simulink model "AUAV3_WITH_SLUGS_SENSOR_AND_CONTROLLER"  (Simulink 8.5)
settings: Solver=FixedStepDiscrete  StartTime=0.0  StopTime=10.0  FixedStep=T  RelTol=1e-3
PreLoadFcn:
  | T = 0.0025;
  | MavlinkBus;
  | 
  | % Baro Altitude Computation
  | % =========================
  | basePressure = 98192.64;
  | baseTemp = 288.215;
  | lapseRate = -0.00198122;
  | baseHeight = 0;
  | 
  | mcuInit
values from neighbouring files (symbols this model uses):
  apSampleTime = 0.01    [mcuInit.m]
  latlong_WP = 1    [mcuInit.m]
  mavlink_gps_raw_int_t = Simulink.Bus    [MavlinkBus.m]    (also in MavlinkBusMarcello.m)
  mavlink_raw_imu_t = Simulink.Bus    [MavlinkBus.m]    (also in MavlinkBusMarcello.m)
  mavlink_scaled_pressure_t = Simulink.Bus    [MavlinkBus.m]    (also in MavlinkBusMarcello.m)
  mavlink_sys_status_t = Simulink.Bus    [MavlinkBus.m]    (also in MavlinkBusMarcello.m)
  Xpoints = [0 0]    [mcuInit.m]
  Ypoints = [0 0]    [mcuInit.m]
  Zpoints = [0 0]    [mcuInit.m]
undefined symbols (not defined in the file or in its folder): A0, A14, A15, A2, A3, A5, A6, accBiasRateLimit, altLatLon, B0, bankCommandLimit, barAdjust, baroCutoff, baroCutTemp, C3, cubeAccelGain16405, cubeGyroGain16405, cubeMagGain16405, D0, D11, D13, D8, daLimit, data, daTrimMax, daTrimMin, deLimit, deTrimMax, deTrimMin, drLimit, drTrimMax, drTrimMin, dtLimit, dtTrimMax, dtTrimMin, F2, F3, G0, G15, gaind, GS_location, gyroBiasRateLimit, IC1max, IPStar, ISA_g, maxAcc, MaxDwnPthStar, maxDynPressure, maxEta, OC1max, P112, P127, P16, P21, P30, P31, P51, P64, P72, P75 ... (+39)
undefined symbols (not defined in the file): baroOffset, baroScale, barTGain1, barTGain2, barTMean1, barTMean2, bda, bde, bdr, bdt, bICda, bICde, bICdr, bICdt, derivativesConstant, lowRateSensorCutoff, mainSensorCutoff, mda, mde, mdr, mdt, mICda, mICde, mICdr, mICdt, pitotOffset, pitotScale, pitTGain1, pitTGain2, pitTMean1, pitTMean2, powerOffset, powerScale, pressureSensorCutoff, tempOffset, tempScale, vzCutoff, xCutoff, yCutoff
libraries: MCHP_Blockset x147, simulink x78, SLUGS_Library x31, aerolibconvert2 x6, aerolibutil x4, aerolibtransform2 x3, dspmtrx3 x2, aerolibobsolete x2
(part 7 of 12)

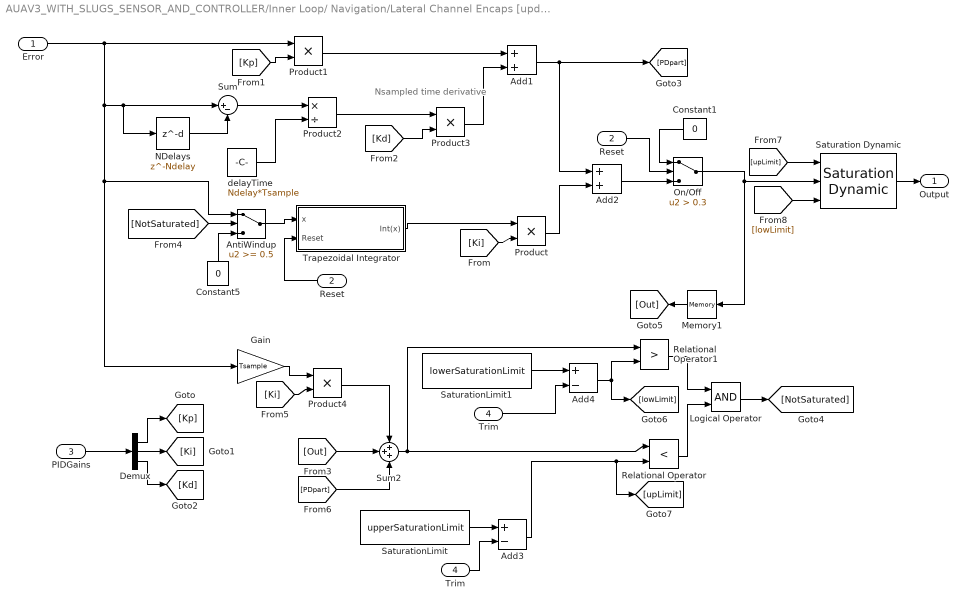
== system AUAV3_WITH_SLUGS_SENSOR_AND_CONTROLLER/Inner Loop/ Navigation/Lateral Channel Encaps [updated 4.28.16]/Lateral Channel/Roll Control [PID] ==
  note: Nsampled time derivative
  Error : Inport
  Reset : Inport  Port=2
  PIDGains : Inport  Port=3
  Trim : Inport  Port=4
  Add1 : Sum
  Add2 : Sum  OutDataTypeStr=single
  Add3 : Sum  Inputs=+-  OutDataTypeStr=single
  Add4 : Sum  Inputs=+-  OutDataTypeStr=single
  AntiWindup : Switch  Threshold=0.5
  Constant1 : Constant  Value=0  OutDataTypeStr=single
  Constant5 : Constant  Value=0  OutDataTypeStr=single
  Demux : Demux  Outputs=3
  Gain : Gain  Gain=Tsample
  Logical Operator : Logic  AllPortsSameDT=off  OutDataTypeStr=boolean
  Memory1 : Memory  InheritSampleTime=on
  NDelays : Delay  DelayLength=Ndelay  InputProcessing=Inherited  SampleTime=Tsample
  On/Off : Switch  Criteria=u2 > Threshold  Threshold=0.3
  Product{,1,3..4} (4 alike) : Product  RndMeth=Zero
  Product2 : Product  Inputs=*/  RndMeth=Zero
  Relational Operator : RelationalOperator  Operator=<  OutDataTypeStr=boolean
  Relational Operator1 : RelationalOperator  Operator=>  OutDataTypeStr=boolean
  "Reset " : InportShadow  Port=2
  Saturation Dynamic : simulink/Discontinuities/Saturation Dynamic  OutMin=[]  OutMax=[]  OutDataTypeStr=Inherit: Same as second input  OutDataType=fixdt(1, 16)  OutScaling=2^-10  DoSatur=off
  SaturationLimit : Constant  Value=upperSaturationLimit  OutDataTypeStr=single
  SaturationLimit1 : Constant  Value=lowerSaturationLimit  OutDataTypeStr=single
  Sum : Sum  Inputs=|+-
  Sum2 : Sum  Inputs=+++
  Trapezoidal Integrator : Subsystem  mask{T=Tsample}
      mask prompts: T "Sample Time"
  "Trim " : InportShadow  Port=4
  delayTime : Constant  Value=Ndelay*Tsample  OutDataTypeStr=single
  Output : Outport
  wires:
  On/Off/1 -> Memory1/1, Saturation Dynamic/2
  Constant1/1 -> On/Off/1
  "Reset "/1 -> On/Off/2
  Add2/1 -> On/Off/3
  [NotSaturated] -> AntiWindup/2
  Saturation Dynamic/1 -> Output/1
  Product2/1 -> Product3/1
  [Kd] -> Product3/2
  delayTime/1 -> Product2/2
  Sum/1 -> Product2/1
  NDelays/1 -> Sum/2
  [Kp] -> Product1/2
  Trapezoidal Integrator/1(Int(x)) -> Product/1
  [Ki] -> Product/2
  Error/1 -> Product1/1, Sum/1, NDelays/1, AntiWindup/1, Gain/1
  AntiWindup/1 -> Trapezoidal Integrator/1(x)
  Constant5/1 -> AntiWindup/3
  Demux/3 -> [Kd]
  Demux/2 -> [Ki]
  Demux/1 -> [Kp]
  PIDGains/1 -> Demux/1
  Memory1/1 -> [Out]
  Reset/1 -> Trapezoidal Integrator/2(Reset)
  Product1/1 -> Add1/1
  Product3/1 -> Add1/2
  Add1/1 -> [PDpart], Add2/1
  Product/1 -> Add2/2
  [PDpart] -> Sum2/3
  Product4/1 -> Sum2/1
  Gain/1 -> Product4/1
  [Ki] -> Product4/2
  Sum2/1 -> Relational Operator/1, Relational Operator1/1
  [Out] -> Sum2/2
  Add3/1 -> Relational Operator/2, [upLimit]
  Relational Operator/1 -> Logical Operator/2
  Relational Operator1/1 -> Logical Operator/1
  Logical Operator/1 -> [NotSaturated]
  Trim/1 -> Add3/2
  SaturationLimit/1 -> Add3/1
  Add4/1 -> Relational Operator1/2, [lowLimit]
  SaturationLimit1/1 -> Add4/1
  "Trim "/1 -> Add4/2
  [upLimit] -> Saturation Dynamic/1
  [lowLimit] -> Saturation Dynamic/3

== system AUAV3_WITH_SLUGS_SENSOR_AND_CONTROLLER/Inner Loop/ Navigation/Lateral Channel Encaps [updated 4.28.16]/Lateral Channel/Sideslip Compensation ==
  phi_m : Inport
  r_m : Inport  Port=2
  U_m : Inport  Port=3
  Enable : EnablePort  StatesWhenEnabling=reset
  Bank to Psi Dot : Subsystem  AncestorBlock=SLUGS_Library/Navigation/Bank to Psi Dot
  Constant : Constant  Value=0.3  OutDataTypeStr=single
  Low Pass : Subsystem
      mask Display:
      | droots([],'-a','a')
      | port_label('input',1,'a')
      | port_label('input',2,'u')
      | port_label('output',1,'y')
  Protect NaNs2 : Subsystem
  Subtract : Sum  Inputs=+-
  psi_dot to Bank : Subsystem  AncestorBlock=SLUGS_Library/Navigation/psi_dot to Bank
  bankComp : Outport  OutputWhenDisabled=reset  InitialOutput=0
  wires:
  Protect NaNs2/1(Out1) -> Low Pass/2(u)
  phi_m/1 -> Bank to Psi Dot/1(phi_c)
  r_m/1 -> Subtract/2
  U_m/1 -> Bank to Psi Dot/2(U_m), psi_dot to Bank/2(U_m)
  Bank to Psi Dot/1(psi_dot_c) -> Subtract/1  "coord turn"
  Subtract/1 -> psi_dot to Bank/1(psi_dot_c)  "turn rate error"
  psi_dot to Bank/1(phi_c) -> Protect NaNs2/1(In1)  "phi error"
  Low Pass/1(y) -> bankComp/1
  Constant/1 -> Low Pass/1(a)

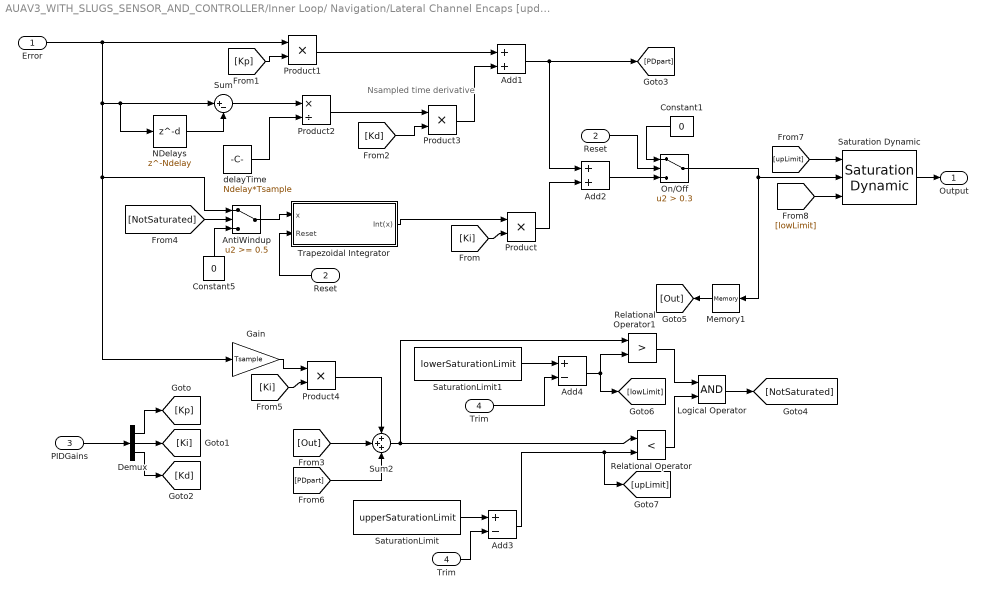
== system AUAV3_WITH_SLUGS_SENSOR_AND_CONTROLLER/Inner Loop/ Navigation/Lateral Channel Encaps [updated 4.28.16]/Lateral Channel/Yaw Damper [PID] ==
  note: Nsampled time derivative
  Error : Inport
  Reset : Inport  Port=2
  PIDGains : Inport  Port=3
  Trim : Inport  Port=4
  Add1 : Sum
  Add2 : Sum  OutDataTypeStr=single
  Add3 : Sum  Inputs=+-  OutDataTypeStr=single
  Add4 : Sum  Inputs=+-  OutDataTypeStr=single
  AntiWindup : Switch  Threshold=0.5
  Constant1 : Constant  Value=0  OutDataTypeStr=single
  Constant5 : Constant  Value=0  OutDataTypeStr=single
  Demux : Demux  Outputs=3
  Gain : Gain  Gain=Tsample
  Logical Operator : Logic  AllPortsSameDT=off  OutDataTypeStr=boolean
  Memory1 : Memory  InheritSampleTime=on
  NDelays : Delay  DelayLength=Ndelay  InputProcessing=Inherited  SampleTime=Tsample
  On/Off : Switch  Criteria=u2 > Threshold  Threshold=0.3
  Product{,1,3..4} (4 alike) : Product  RndMeth=Zero
  Product2 : Product  Inputs=*/  RndMeth=Zero
  Relational Operator : RelationalOperator  Operator=<  OutDataTypeStr=boolean
  Relational Operator1 : RelationalOperator  Operator=>  OutDataTypeStr=boolean
  "Reset " : InportShadow  Port=2
  Saturation Dynamic : simulink/Discontinuities/Saturation Dynamic  OutMin=[]  OutMax=[]  OutDataTypeStr=Inherit: Same as second input  OutDataType=fixdt(1, 16)  OutScaling=2^-10  DoSatur=off
  SaturationLimit : Constant  Value=upperSaturationLimit  OutDataTypeStr=single
  SaturationLimit1 : Constant  Value=lowerSaturationLimit  OutDataTypeStr=single
  Sum : Sum  Inputs=|+-
  Sum2 : Sum  Inputs=+++
  Trapezoidal Integrator : Subsystem  mask{T=Tsample}
      mask prompts: T "Sample Time"
  "Trim " : InportShadow  Port=4
  delayTime : Constant  Value=Ndelay*Tsample  OutDataTypeStr=single
  Output : Outport
  wires:
  On/Off/1 -> Memory1/1, Saturation Dynamic/2
  Constant1/1 -> On/Off/1
  "Reset "/1 -> On/Off/2
  Add2/1 -> On/Off/3
  [NotSaturated] -> AntiWindup/2
  Saturation Dynamic/1 -> Output/1
  Product2/1 -> Product3/1
  [Kd] -> Product3/2
  delayTime/1 -> Product2/2
  Sum/1 -> Product2/1
  NDelays/1 -> Sum/2
  [Kp] -> Product1/2
  Trapezoidal Integrator/1(Int(x)) -> Product/1
  [Ki] -> Product/2
  Error/1 -> Product1/1, Sum/1, NDelays/1, AntiWindup/1, Gain/1
  AntiWindup/1 -> Trapezoidal Integrator/1(x)
  Constant5/1 -> AntiWindup/3
  Demux/3 -> [Kd]
  Demux/2 -> [Ki]
  Demux/1 -> [Kp]
  PIDGains/1 -> Demux/1
  Memory1/1 -> [Out]
  Reset/1 -> Trapezoidal Integrator/2(Reset)
  Product1/1 -> Add1/1
  Product3/1 -> Add1/2
  Add1/1 -> [PDpart], Add2/1
  Product/1 -> Add2/2
  [PDpart] -> Sum2/3
  Product4/1 -> Sum2/1
  Gain/1 -> Product4/1
  [Ki] -> Product4/2
  Sum2/1 -> Relational Operator/1, Relational Operator1/1
  [Out] -> Sum2/2
  Add3/1 -> Relational Operator/2, [upLimit]
  Relational Operator/1 -> Logical Operator/2
  Relational Operator1/1 -> Logical Operator/1
  Logical Operator/1 -> [NotSaturated]
  Trim/1 -> Add3/2
  SaturationLimit/1 -> Add3/1
  Add4/1 -> Relational Operator1/2, [lowLimit]
  SaturationLimit1/1 -> Add4/1
  "Trim "/1 -> Add4/2
  [upLimit] -> Saturation Dynamic/1
  [lowLimit] -> Saturation Dynamic/3

== system AUAV3_WITH_SLUGS_SENSOR_AND_CONTROLLER/Inner Loop/ Navigation/Lateral Channel Encaps [updated 4.28.16]/Lateral Channel/psi_dot to Bank ==
  psi_dot_c : Inport
  U_m : Inport  Port=2
  Constant1 : Constant  Value=9.80665  OutDataTypeStr=single
  Divide : Product  Inputs=**/
  dsPIC_atan : Subsystem  AncestorBlock=SLUGS_Library/dsPIC_atan
  phi_c : Outport
  wires:
  Divide/1 -> dsPIC_atan/1(x)
  dsPIC_atan/1(atan(x)) -> phi_c/1
  Constant1/1 -> Divide/3
  U_m/1 -> Divide/2
  psi_dot_c/1 -> Divide/1

== system AUAV3_WITH_SLUGS_SENSOR_AND_CONTROLLER/Inner Loop/ Navigation/Lateral Channel Encaps [updated 4.28.16]/psi_dot_c Select logic1/Bank to Psi Dot ==
  phi_c : Inport
  U_m : Inport  Port=2
  Constant1 : Constant  Value=9.80665  OutDataTypeStr=single
  Divide : Product  Inputs=/*  OutDataTypeStr=single
  Divide1 : Product  OutDataTypeStr=single
  Protect NaNs : Subsystem
  Protect NaNs1 : Subsystem
  "[0 40]" : Saturate  UpperLimit=40  LowerLimit=0  SampleTime=.01
  bank Limit : Saturate  UpperLimit=bankCommandLimit  LowerLimit=-bankCommandLimit  SampleTime=.01
  dsPIC_tan : Subsystem  AncestorBlock=SLUGS_Library/dsPIC_tan
  psi_dot_c : Outport
  wires:
  "[0 40]"/1 -> Divide/1
  Divide/1 -> Divide1/2
  phi_c/1 -> Protect NaNs/1(In1)
  dsPIC_tan/1(tan(x)) -> Divide1/1
  Divide1/1 -> psi_dot_c/1
  Constant1/1 -> Divide/2
  U_m/1 -> Protect NaNs1/1(In1)
  bank Limit/1 -> dsPIC_tan/1(x)
  Protect NaNs/1(Out1) -> bank Limit/1
  Protect NaNs1/1(Out1) -> "[0 40]"/1

== system AUAV3_WITH_SLUGS_SENSOR_AND_CONTROLLER/Inner Loop/ Navigation/Longitudinal Channel Encaps [updated 4.28.16]/Longitudinal Channel/0.5 sec  tau for Turns ==
  In1 : Inport
  Constant : Constant  Value=T
  Constant1 : Constant  Value=f
  Embedded MATLAB Function : MATLAB Function  TreatAsAtomicUnit=on
  Out1 : Outport
  wires:
  Constant/1 -> Embedded MATLAB Function/2(T)
  Constant1/1 -> Embedded MATLAB Function/3(f)
  Embedded MATLAB Function/1(y) -> Out1/1
  In1/1 -> Embedded MATLAB Function/1(u)

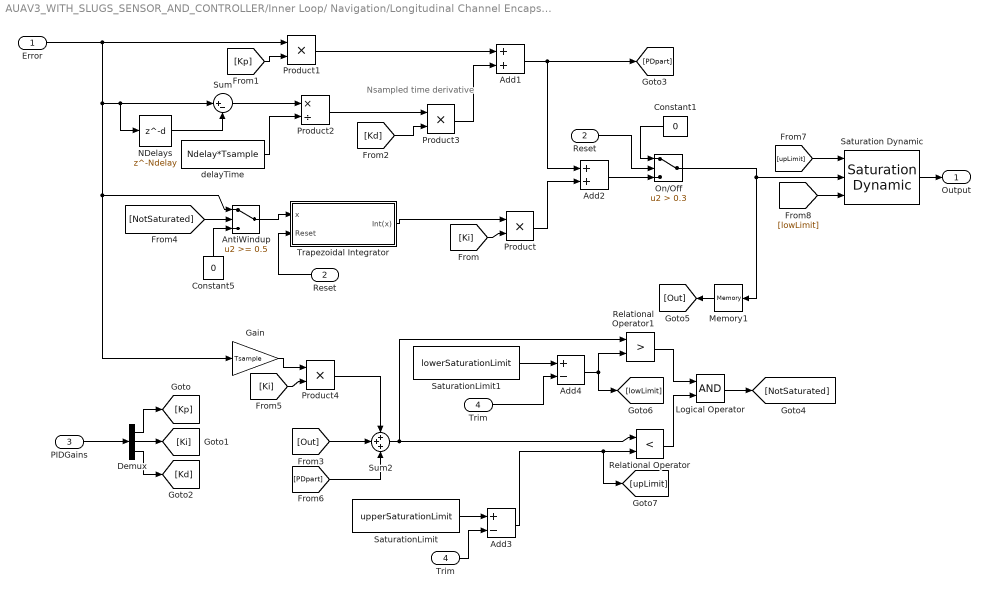
== system AUAV3_WITH_SLUGS_SENSOR_AND_CONTROLLER/Inner Loop/ Navigation/Longitudinal Channel Encaps [updated 4.28.16]/Longitudinal Channel/Airspeed Hold [PID] ==
  note: Nsampled time derivative
  Error : Inport
  Reset : Inport  Port=2
  PIDGains : Inport  Port=3
  Trim : Inport  Port=4
  Add1 : Sum
  Add2 : Sum  OutDataTypeStr=single
  Add3 : Sum  Inputs=+-  OutDataTypeStr=single
  Add4 : Sum  Inputs=+-  OutDataTypeStr=single
  AntiWindup : Switch  Threshold=0.5
  Constant1 : Constant  Value=0  OutDataTypeStr=single
  Constant5 : Constant  Value=0  OutDataTypeStr=single
  Demux : Demux  Outputs=3
  Gain : Gain  Gain=Tsample
  Logical Operator : Logic  AllPortsSameDT=off  OutDataTypeStr=boolean
  Memory1 : Memory  InheritSampleTime=on
  NDelays : Delay  DelayLength=Ndelay  InputProcessing=Inherited  SampleTime=Tsample
  On/Off : Switch  Criteria=u2 > Threshold  Threshold=0.3
  Product{,1,3..4} (4 alike) : Product  RndMeth=Zero
  Product2 : Product  Inputs=*/  RndMeth=Zero
  Relational Operator : RelationalOperator  Operator=<  OutDataTypeStr=boolean
  Relational Operator1 : RelationalOperator  Operator=>  OutDataTypeStr=boolean
  "Reset " : InportShadow  Port=2
  Saturation Dynamic : simulink/Discontinuities/Saturation Dynamic  OutMin=[]  OutMax=[]  OutDataTypeStr=Inherit: Same as second input  OutDataType=fixdt(1, 16)  OutScaling=2^-10  DoSatur=off
  SaturationLimit : Constant  Value=upperSaturationLimit  OutDataTypeStr=single
  SaturationLimit1 : Constant  Value=lowerSaturationLimit  OutDataTypeStr=single
  Sum : Sum  Inputs=|+-
  Sum2 : Sum  Inputs=+++
  Trapezoidal Integrator : Subsystem  mask{T=Tsample}
      mask prompts: T "Sample Time"
  "Trim " : InportShadow  Port=4
  delayTime : Constant  Value=Ndelay*Tsample  OutDataTypeStr=single
  Output : Outport
  wires:
  On/Off/1 -> Memory1/1, Saturation Dynamic/2
  Constant1/1 -> On/Off/1
  "Reset "/1 -> On/Off/2
  Add2/1 -> On/Off/3
  [NotSaturated] -> AntiWindup/2
  Saturation Dynamic/1 -> Output/1
  Product2/1 -> Product3/1
  [Kd] -> Product3/2
  delayTime/1 -> Product2/2
  Sum/1 -> Product2/1
  NDelays/1 -> Sum/2
  [Kp] -> Product1/2
  Trapezoidal Integrator/1(Int(x)) -> Product/1
  [Ki] -> Product/2
  Error/1 -> Product1/1, Sum/1, NDelays/1, AntiWindup/1, Gain/1
  AntiWindup/1 -> Trapezoidal Integrator/1(x)
  Constant5/1 -> AntiWindup/3
  Demux/3 -> [Kd]
  Demux/2 -> [Ki]
  Demux/1 -> [Kp]
  PIDGains/1 -> Demux/1
  Memory1/1 -> [Out]
  Reset/1 -> Trapezoidal Integrator/2(Reset)
  Product1/1 -> Add1/1
  Product3/1 -> Add1/2
  Add1/1 -> [PDpart], Add2/1
  Product/1 -> Add2/2
  [PDpart] -> Sum2/3
  Product4/1 -> Sum2/1
  Gain/1 -> Product4/1
  [Ki] -> Product4/2
  Sum2/1 -> Relational Operator/1, Relational Operator1/1
  [Out] -> Sum2/2
  Add3/1 -> Relational Operator/2, [upLimit]
  Relational Operator/1 -> Logical Operator/2
  Relational Operator1/1 -> Logical Operator/1
  Logical Operator/1 -> [NotSaturated]
  Trim/1 -> Add3/2
  SaturationLimit/1 -> Add3/1
  Add4/1 -> Relational Operator1/2, [lowLimit]
  SaturationLimit1/1 -> Add4/1
  "Trim "/1 -> Add4/2
  [upLimit] -> Saturation Dynamic/1
  [lowLimit] -> Saturation Dynamic/3

== system AUAV3_WITH_SLUGS_SENSOR_AND_CONTROLLER/Inner Loop/ Navigation/Longitudinal Channel Encaps [updated 4.28.16]/Longitudinal Channel/Height Error to Pitch  Command [PI] ==
  Error : Inport
  Reset : Inport  Port=2
  PIDGains : Inport  Port=3
  Trim : Inport  Port=4
  Add2 : Sum  OutDataTypeStr=single
  Add3 : Sum  Inputs=+-  OutDataTypeStr=single
  Add4 : Sum  Inputs=+-  OutDataTypeStr=single
  AntiWindup : Switch  Threshold=0.5
  Constant1 : Constant  Value=0  OutDataTypeStr=single
  Constant5 : Constant  Value=0  OutDataTypeStr=single
  Demux : Demux  Outputs=3
  Gain : Gain  Gain=Tsample
  Logical Operator : Logic  AllPortsSameDT=off  OutDataTypeStr=boolean
  Memory1 : Memory  InheritSampleTime=on
  On/Off : Switch  Criteria=u2 > Threshold  Threshold=0.3
  Product : Product  RndMeth=Zero
  Product1 : Product  RndMeth=Zero
  Product4 : Product  RndMeth=Zero
  Relational Operator : RelationalOperator  Operator=<  OutDataTypeStr=boolean
  Relational Operator1 : RelationalOperator  Operator=>  OutDataTypeStr=boolean
  "Reset " : InportShadow  Port=2
  Saturation Dynamic : simulink/Discontinuities/Saturation Dynamic  OutMin=[]  OutMax=[]  OutDataTypeStr=Inherit: Same as second input  OutDataType=fixdt(1, 16)  OutScaling=2^-10  DoSatur=off
  SaturationLimit : Constant  Value=upperSaturationLimit  OutDataTypeStr=single
  SaturationLimit1 : Constant  Value=lowerSaturationLimit  OutDataTypeStr=single
  Sum2 : Sum  Inputs=+++
  Terminator3 : Terminator
  Trapezoidal Integrator : Subsystem  mask{T=Tsample}
      mask prompts: T "Sample Time"
  "Trim " : InportShadow  Port=4
  Output : Outport
  wires:
  On/Off/1 -> Memory1/1, Saturation Dynamic/2
  Constant1/1 -> On/Off/1
  "Reset "/1 -> On/Off/2
  Add2/1 -> On/Off/3
  [lowLimit] -> Saturation Dynamic/3
  [upLimit] -> Saturation Dynamic/1
  "Trim "/1 -> Add4/2
  SaturationLimit1/1 -> Add4/1
  Add4/1 -> [lowLimit], Relational Operator1/2
  SaturationLimit/1 -> Add3/1
  Trim/1 -> Add3/2
  Logical Operator/1 -> [NotSaturated]
  Relational Operator1/1 -> Logical Operator/1
  Relational Operator/1 -> Logical Operator/2
  Add3/1 -> [upLimit], Relational Operator/2
  [Out] -> Sum2/2
  Sum2/1 -> Relational Operator1/1, Relational Operator/1
  [Ki] -> Product4/2
  Gain/1 -> Product4/1
  Product4/1 -> Sum2/1
  [PDpart] -> Sum2/3
  Product/1 -> Add2/2
  Product1/1 -> Add2/1, [PDpart]
  Reset/1 -> Trapezoidal Integrator/2(Reset)
  Memory1/1 -> [Out]
  PIDGains/1 -> Demux/1
  Demux/1 -> [Kp]
  Demux/2 -> [Ki]
  Constant5/1 -> AntiWindup/3
  AntiWindup/1 -> Trapezoidal Integrator/1(x)
  Error/1 -> Product1/1, Gain/1, AntiWindup/1
  [Ki] -> Product/2
  Trapezoidal Integrator/1(Int(x)) -> Product/1
  [Kp] -> Product1/2
  Saturation Dynamic/1 -> Output/1
  [NotSaturated] -> AntiWindup/2
  Demux/3 -> Terminator3/1

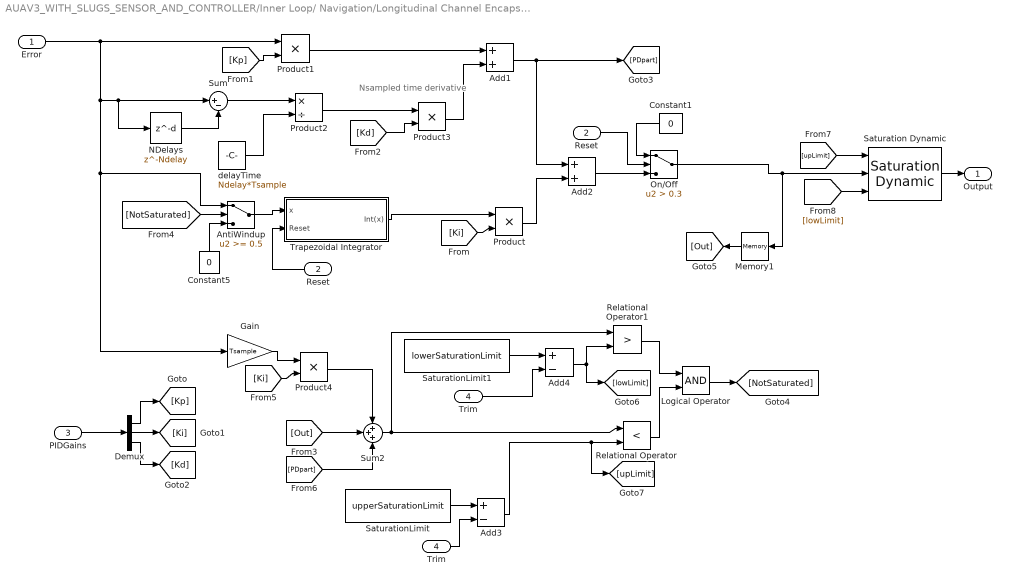
== system AUAV3_WITH_SLUGS_SENSOR_AND_CONTROLLER/Inner Loop/ Navigation/Longitudinal Channel Encaps [updated 4.28.16]/Longitudinal Channel/Pitch To Elevator [PID] ==
  note: Nsampled time derivative
  Error : Inport
  Reset : Inport  Port=2
  PIDGains : Inport  Port=3
  Trim : Inport  Port=4
  Add1 : Sum
  Add2 : Sum  OutDataTypeStr=single
  Add3 : Sum  Inputs=+-  OutDataTypeStr=single
  Add4 : Sum  Inputs=+-  OutDataTypeStr=single
  AntiWindup : Switch  Threshold=0.5
  Constant1 : Constant  Value=0  OutDataTypeStr=single
  Constant5 : Constant  Value=0  OutDataTypeStr=single
  Demux : Demux  Outputs=3
  Gain : Gain  Gain=Tsample
  Logical Operator : Logic  AllPortsSameDT=off  OutDataTypeStr=boolean
  Memory1 : Memory  InheritSampleTime=on
  NDelays : Delay  DelayLength=Ndelay  InputProcessing=Inherited  SampleTime=Tsample
  On/Off : Switch  Criteria=u2 > Threshold  Threshold=0.3
  Product{,1,3..4} (4 alike) : Product  RndMeth=Zero
  Product2 : Product  Inputs=*/  RndMeth=Zero
  Relational Operator : RelationalOperator  Operator=<  OutDataTypeStr=boolean
  Relational Operator1 : RelationalOperator  Operator=>  OutDataTypeStr=boolean
  "Reset " : InportShadow  Port=2
  Saturation Dynamic : simulink/Discontinuities/Saturation Dynamic  OutMin=[]  OutMax=[]  OutDataTypeStr=Inherit: Same as second input  OutDataType=fixdt(1, 16)  OutScaling=2^-10  DoSatur=off
  SaturationLimit : Constant  Value=upperSaturationLimit  OutDataTypeStr=single
  SaturationLimit1 : Constant  Value=lowerSaturationLimit  OutDataTypeStr=single
  Sum : Sum  Inputs=|+-
  Sum2 : Sum  Inputs=+++
  Trapezoidal Integrator : Subsystem  mask{T=Tsample}
      mask prompts: T "Sample Time"
  "Trim " : InportShadow  Port=4
  delayTime : Constant  Value=Ndelay*Tsample  OutDataTypeStr=single
  Output : Outport
  wires:
  On/Off/1 -> Memory1/1, Saturation Dynamic/2
  Constant1/1 -> On/Off/1
  "Reset "/1 -> On/Off/2
  Add2/1 -> On/Off/3
  [NotSaturated] -> AntiWindup/2
  Saturation Dynamic/1 -> Output/1
  Product2/1 -> Product3/1
  [Kd] -> Product3/2
  delayTime/1 -> Product2/2
  Sum/1 -> Product2/1
  NDelays/1 -> Sum/2
  [Kp] -> Product1/2
  Trapezoidal Integrator/1(Int(x)) -> Product/1
  [Ki] -> Product/2
  Error/1 -> Product1/1, Sum/1, NDelays/1, AntiWindup/1, Gain/1
  AntiWindup/1 -> Trapezoidal Integrator/1(x)
  Constant5/1 -> AntiWindup/3
  Demux/3 -> [Kd]
  Demux/2 -> [Ki]
  Demux/1 -> [Kp]
  PIDGains/1 -> Demux/1
  Memory1/1 -> [Out]
  Reset/1 -> Trapezoidal Integrator/2(Reset)
  Product1/1 -> Add1/1
  Product3/1 -> Add1/2
  Add1/1 -> [PDpart], Add2/1
  Product/1 -> Add2/2
  [PDpart] -> Sum2/3
  Product4/1 -> Sum2/1
  Gain/1 -> Product4/1
  [Ki] -> Product4/2
  Sum2/1 -> Relational Operator/1, Relational Operator1/1
  [Out] -> Sum2/2
  Add3/1 -> Relational Operator/2, [upLimit]
  Relational Operator/1 -> Logical Operator/2
  Relational Operator1/1 -> Logical Operator/1
  Logical Operator/1 -> [NotSaturated]
  Trim/1 -> Add3/2
  SaturationLimit/1 -> Add3/1
  Add4/1 -> Relational Operator1/2, [lowLimit]
  SaturationLimit1/1 -> Add4/1
  "Trim "/1 -> Add4/2
  [upLimit] -> Saturation Dynamic/1
  [lowLimit] -> Saturation Dynamic/3

== system AUAV3_WITH_SLUGS_SENSOR_AND_CONTROLLER/Inner Loop/ Navigation/Longitudinal Channel Encaps [updated 4.28.16]/Longitudinal Channel/Pitot Control End ==
  dyn P [Pa] : Inport
  H_m [m] : Inport  Port=2
  " 0.3 sec tau for high speeds" : Subsystem  mask(Tustin1stOrderLowpassAutoInitialCondition){f=1, T=T}
      mask prompts: f "Lowpass Frequency"; T "Sample Time"
      mask help: Takes a 3db rolloff frequency (in Hz, NOT radians/s) and a sample time. Performs a symbolic Tustin conversion and implements in a discrete filter. The initial output of the filter is set by the first sample.
      mask Help: Enter the desired 3db rolloff frequency in Hz and the sample time. Initial conditions are sampled automatically.
      mask Display: fprintf('%.2f Hz lowpass',f)
  Air Density from Height : Subsystem
  Compute Airspeed : Subsystem
  Protect NaN : Subsystem
  Schedule LPF : Switch  Criteria=u2 > Threshold  Threshold=0.3  OutDataTypeStr=single
  lowpass limit : simulink/Logic and Bit Operations/Compare To Constant  relop=<=  const=5  OutDataTypeStr=uint8  ZeroCross=off
  AirSpeed[m/s] : Outport
  wires:
  H_m [m]/1 -> Air Density from Height/1(h(m))
  Schedule LPF/1 -> AirSpeed[m/s]/1
  dyn P [Pa]/1 -> Compute Airspeed/1(Dyn P)
  Air Density from Height/1(rho (Kg/m^3)) -> Compute Airspeed/2(rho)
  Compute Airspeed/1(Airspeed m(s)) -> Protect NaN/1(In1)
  lowpass limit/1 -> Schedule LPF/2
  " 0.3 sec tau for high speeds"/1(Out1) -> Schedule LPF/3
  Protect NaN/1(Out1) -> " 0.3 sec tau for high speeds"/1(In1), lowpass limit/1, Schedule LPF/1

== system AUAV3_WITH_SLUGS_SENSOR_AND_CONTROLLER/Inner Loop/ Navigation/Longitudinal Channel Encaps [updated 4.28.16]/Longitudinal Channel/Protect NaNs ==
  In1 : Inport
  Integer Delay3 : Delay  DelayLength=1  InputProcessing=Inherited  SampleTime=T
  Relational Operator2 : RelationalOperator  Operator===  OutDataTypeStr=uint(8)
  Switch3 : Switch  Criteria=u2 > Threshold  Threshold=0.3  SampleTime=.01
  Out1 : Outport
  wires:
  Integer Delay3/1 -> Switch3/3
  Switch3/1 -> Out1/1, Integer Delay3/1
  In1/1 -> Relational Operator2/2, Relational Operator2/1, Switch3/1
  Relational Operator2/1 -> Switch3/2

== system AUAV3_WITH_SLUGS_SENSOR_AND_CONTROLLER/Inner Loop/ Navigation/Longitudinal Channel Encaps [updated 4.28.16]/Longitudinal Channel/Protect NaNs1 ==
  In1 : Inport
  Integer Delay3 : Delay  DelayLength=1  InputProcessing=Inherited  SampleTime=T
  Relational Operator2 : RelationalOperator  Operator===  OutDataTypeStr=uint(8)
  Switch3 : Switch  Criteria=u2 > Threshold  Threshold=0.3  SampleTime=.01
  Out1 : Outport
  wires:
  Integer Delay3/1 -> Switch3/3
  Switch3/1 -> Out1/1, Integer Delay3/1
  In1/1 -> Relational Operator2/2, Relational Operator2/1, Switch3/1
  Relational Operator2/1 -> Switch3/2

== system AUAV3_WITH_SLUGS_SENSOR_AND_CONTROLLER/Inner Loop/ Navigation/Longitudinal Channel Encaps [updated 4.28.16]/Longitudinal Channel/Protect NaNs2 ==
  In1 : Inport
  Integer Delay3 : Delay  DelayLength=1  InputProcessing=Inherited  SampleTime=T
  Relational Operator2 : RelationalOperator  Operator===  OutDataTypeStr=uint(8)
  Switch3 : Switch  Criteria=u2 > Threshold  Threshold=0.3  SampleTime=.01
  Out1 : Outport
  wires:
  Relational Operator2/1 -> Switch3/2
  In1/1 -> Switch3/1, Relational Operator2/1, Relational Operator2/2
  Switch3/1 -> Integer Delay3/1, Out1/1
  Integer Delay3/1 -> Switch3/3

== system AUAV3_WITH_SLUGS_SENSOR_AND_CONTROLLER/Inner Loop/ Navigation/Longitudinal Channel Encaps [updated 4.28.16]/Longitudinal Channel/Protect NaNs4 ==
  In1 : Inport
  Integer Delay3 : Delay  DelayLength=1  InputProcessing=Inherited  SampleTime=T
  Relational Operator2 : RelationalOperator  Operator===  OutDataTypeStr=uint(8)
  Switch3 : Switch  Criteria=u2 > Threshold  Threshold=0.3  SampleTime=.01
  Out1 : Outport
  wires:
  Relational Operator2/1 -> Switch3/2
  In1/1 -> Switch3/1, Relational Operator2/1, Relational Operator2/2
  Switch3/1 -> Integer Delay3/1, Out1/1
  Integer Delay3/1 -> Switch3/3

== system AUAV3_WITH_SLUGS_SENSOR_AND_CONTROLLER/Inner Loop/ Navigation/Longitudinal Channel Encaps [updated 4.28.16]/Longitudinal Channel/dsPIC_cos ==
  u : Inport
  Environment Controller1 : simulink/Signal Routing/Environment Controller
  Trigonometric Function : Trigonometry  Operator=cos
  myCos() apUtils.c [updated 5.1.16] : MCHP_Blockset/User Functions/C Function Call  ParseFilesChkbx=off  ListFunctions1=Custom Function  Function1=float myCos(float x)  AddHeaderDeclaration=off  Function1Type=when block is updated (default)  Fct1BlockIn=x  FctReturnBlockOut=on  DataCollected=0  ORDERING=None  SampleTime=-1  MCHP_MASTERLINK=|  PinDigitalInput=[]  PinDigitalOutput=[]  PinAnalogInput=[]
      | AUAV3_WITH_SLUGS_SENSOR_AND_CONTROLLER/Microchip Master
      | AUAV V3 Board
      | Busy Flag on D2 (RA6)
  cos(u) : Outport
  wires:
  u/1 -> Trigonometric Function/1, myCos() apUtils.c [updated 5.1.16]/1
  Environment Controller1/1 -> cos(u)/1
  myCos() apUtils.c [updated 5.1.16]/1 -> Environment Controller1/2
  Trigonometric Function/1 -> Environment Controller1/1

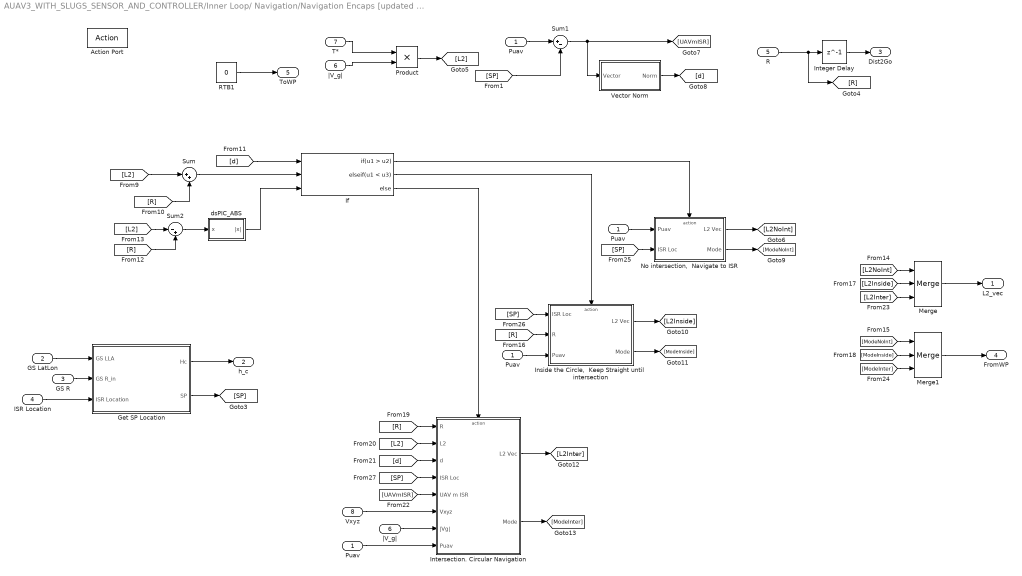
== system AUAV3_WITH_SLUGS_SENSOR_AND_CONTROLLER/Inner Loop/ Navigation/Navigation Encaps [updated 4.28.16]/Navigation/Circle Navigation ==
  Puav : Inport
  GS LatLon : Inport  Port=2
  GS R : Inport  Port=3
  ISR Location : Inport  Port=4
  R : Inport  Port=5
  |V_g| : Inport  Port=6
  T* : Inport  Port=7
  Vxyz : Inport  Port=8
  Action Port : ActionPort  ActionType=elseif
  Get SP Location : Subsystem
  If : If  NumInputs=3  IfExpression=u1 > u2  ElseIfExpressions=u1 < u3
  "Inside the Circle,  Keep Straight until  intersection" : Subsystem  TreatAsAtomicUnit=on
  Integer Delay : Delay  DelayLength=1  InputProcessing=Inherited
  Intersection. Circular Navigation : Subsystem  TreatAsAtomicUnit=on
  Merge : Merge  Inputs=3
  Merge1 : Merge  Inputs=3
  "No intersection,  Navigate to ISR" : Subsystem  TreatAsAtomicUnit=on
  Product : Product  OutDataTypeStr=single  RndMeth=Zero
  "Puav   " : InportShadow
  "Puav    " : InportShadow
  "Puav     " : InportShadow
  RTB1 : Constant  Value=0  OutDataTypeStr=uint8
  Sum : Sum  Inputs=|++
  Sum1 : Sum  Inputs=|+-
  Sum2 : Sum  Inputs=|-+
  Vector Norm : Subsystem  AncestorBlock=SLUGS_Library/Vector Norm
  dsPIC_ABS : Subsystem  AncestorBlock=SLUGS_Library/dsPIC_ABS
  "|V_g| " : InportShadow  Port=6
  L2_vec : Outport
  h_c : Outport  Port=2
  Dist2Go : Outport  Port=3
  FromWP : Outport  Port=4  InitialOutput=[1]
  ToWP : Outport  Port=5  InitialOutput=[1]
  wires:
  Merge1/1 -> FromWP/1
  R/1 -> [R], Integer Delay/1
  Integer Delay/1 -> Dist2Go/1
  ISR Location/1 -> Get SP Location/3(ISR Location)
  GS R/1 -> Get SP Location/2(GS R_in)
  GS LatLon/1 -> Get SP Location/1(GS LLA)
  Get SP Location/2(SP) -> [SP]
  Product/1 -> [L2]
  |V_g|/1 -> Product/2
  T*/1 -> Product/1
  RTB1/1 -> ToWP/1
  [L2] -> Sum/1
  [R] -> Sum/2
  "Puav   "/1 -> Sum1/1
  [SP] -> Sum1/2
  Sum1/1 -> Vector Norm/1(Vector), [UAVmISR]
  Vector Norm/1(Norm) -> [d]
  [d] -> If/1
  Sum/1 -> If/2
  [L2] -> Sum2/1
  [R] -> Sum2/2
  Sum2/1 -> dsPIC_ABS/1(x)
  dsPIC_ABS/1(|x|) -> If/3
  Merge/1 -> L2_vec/1
  If/1 -> "No intersection,  Navigate to ISR"/Action
  If/2 -> "Inside the Circle,  Keep Straight until  intersection"/Action
  If/3 -> Intersection. Circular Navigation/Action
  "Puav    "/1 -> "No intersection,  Navigate to ISR"/1(Puav)
  [SP] -> "No intersection,  Navigate to ISR"/2(ISR Loc)
  "No intersection,  Navigate to ISR"/1(L2 Vec) -> [L2NoInt]
  "No intersection,  Navigate to ISR"/2(Mode) -> [ModeNoInt]
  [L2NoInt] -> Merge/1
  [ModeNoInt] -> Merge1/1
  [SP] -> "Inside the Circle,  Keep Straight until  intersection"/1(ISR Loc)
  [R] -> "Inside the Circle,  Keep Straight until  intersection"/2(R)
  "Inside the Circle,  Keep Straight until  intersection"/1(L2 Vec) -> [L2Inside]
  "Inside the Circle,  Keep Straight until  intersection"/2(Mode) -> [ModeInside]
  [L2Inside] -> Merge/2
  [ModeInside] -> Merge1/2
  Puav/1 -> "Inside the Circle,  Keep Straight until  intersection"/3(Puav)
  Intersection. Circular Navigation/1(L2 Vec) -> [L2Inter]
  Intersection. Circular Navigation/2(Mode) -> [ModeInter]
  [R] -> Intersection. Circular Navigation/1(R)
  [L2] -> Intersection. Circular Navigation/2(L2)
  [d] -> Intersection. Circular Navigation/3(d)
  [SP] -> Intersection. Circular Navigation/4(ISR Loc)
  [UAVmISR] -> Intersection. Circular Navigation/5(UAV m ISR)
  Vxyz/1 -> Intersection. Circular Navigation/6(Vxyz)
  "|V_g| "/1 -> Intersection. Circular Navigation/7(|Vg|)
  [L2Inter] -> Merge/3
  [ModeInter] -> Merge1/3
  Get SP Location/1(Hc) -> h_c/1
  "Puav     "/1 -> Intersection. Circular Navigation/8(Puav)

== system AUAV3_WITH_SLUGS_SENSOR_AND_CONTROLLER/Inner Loop/ Navigation/Navigation Encaps [updated 4.28.16]/Navigation/Get 2D Groundspeed ==
  Vxyz : Inport  SampleTime=apSampleTime
  Vector Norm : Subsystem  AncestorBlock=SLUGS_Library/Vector Norm
  |V_g| : Outport
  wires:
  Vxyz/1 -> Vector Norm/1(Vector)
  Vector Norm/1(Norm) -> |V_g|/1

== system AUAV3_WITH_SLUGS_SENSOR_AND_CONTROLLER/Inner Loop/ Navigation/Navigation Encaps [updated 4.28.16]/Navigation/L2+ ==
  |V_g| : Inport
  L2_vec : Inport  Port=2
  Vxyz : Inport  Port=3
  T*(m) : Inport  Port=4
  Constant10 : Constant  Value=maxEta  OutDataTypeStr=single
  "Get Sin, Cos eta" : Subsystem
  L2+ : Subsystem
  Rad2Deg : Gain  Gain=180/pi
  Relational Operator : RelationalOperator  Operator=<=  OutDataTypeStr=boolean
  Subsystem : Subsystem
  Switch : Switch  Criteria=u2 > Threshold  Threshold=0.3
  dsPIC_ABS : Subsystem  AncestorBlock=SLUGS_Library/dsPIC_ABS
  dsPIC_atan2 : Subsystem  AncestorBlock=SLUGS_Library/dsPIC_atan2
  "if sin(eta) < 0 - maxAcc else                 maxAcc " : Subsystem
  "|V_g| " : InportShadow
  phi_c : Outport
  eta : Outport  Port=2
  wires:
  Vxyz/1 -> "Get Sin, Cos eta"/3(Vxyz)
  L2_vec/1 -> "Get Sin, Cos eta"/2(L2_vec)
  |V_g|/1 -> "Get Sin, Cos eta"/1(|V_g|)
  Switch/1 -> Subsystem/1(a_c)
  "if sin(eta) < 0 - maxAcc else                 maxAcc "/1(+ - maxAcc) -> Switch/3
  L2+/1(a_c) -> Switch/1
  Relational Operator/1 -> Switch/2
  Constant10/1 -> Relational Operator/2
  dsPIC_ABS/1(|x|) -> Relational Operator/1
  dsPIC_atan2/1(atan2(x,y)) -> dsPIC_ABS/1(x), Rad2Deg/1  "eta"
  "Get Sin, Cos eta"/2(cos(eta)) -> dsPIC_atan2/2(v)
  "Get Sin, Cos eta"/1(sin(eta)) -> "if sin(eta) < 0 - maxAcc else                 maxAcc "/1(sin(eta)), dsPIC_atan2/1(u), L2+/1(sin(eta))
  "|V_g| "/1 -> L2+/2(|V_g|)
  T*(m)/1 -> L2+/3(T*)
  Subsystem/1(phi_c) -> phi_c/1
  Rad2Deg/1 -> eta/1

== system AUAV3_WITH_SLUGS_SENSOR_AND_CONTROLLER/Inner Loop/ Navigation/Navigation Encaps [updated 4.28.16]/Navigation/Line Segment ==
  Puav : Inport
  MidLvl h_c : Inport  Port=2
  Action Port : ActionPort  ActionType=elseif
  Gain : Gain  Gain=-1
  Gain1 : Gain  Gain=-1
  "Puav " : InportShadow
  RTB : Constant  Value=0  OutDataTypeStr=uint8
  RTB1 : Constant  Value=0  OutDataTypeStr=uint8
  Vector Norm : Subsystem  AncestorBlock=SLUGS_Library/Vector Norm
  L2_vec : Outport
  h_c : Outport  Port=2
  Dist2Go : Outport  Port=3
  FromWP : Outport  Port=4  InitialOutput=[1]
  ToWP : Outport  Port=5  InitialOutput=[2]
  wires:
  RTB1/1 -> ToWP/1
  Gain1/1 -> Vector Norm/1(Vector)
  "Puav "/1 -> Gain1/1
  RTB/1 -> FromWP/1
  Vector Norm/1(Norm) -> Dist2Go/1
  MidLvl h_c/1 -> h_c/1
  Puav/1 -> Gain/1
  Gain/1 -> L2_vec/1

== system AUAV3_WITH_SLUGS_SENSOR_AND_CONTROLLER/Inner Loop/ Navigation/Navigation Encaps [updated 4.28.16]/Navigation/Minimum Turn Radius ==
  U_c : Inport
  Scale Factor : Inport  Port=2
  Constant1 : Constant  Value=maxAcc  OutDataTypeStr=single
  IC : InitialCondition  Value=1.5
  Product1 : Product  RndMeth=Zero
  Product2 : Product  RndMeth=Zero
  Product3 : Product  Inputs=*/  RndMeth=Zero
  "[1.5 10]" : Saturate  UpperLimit=10  LowerLimit=1.5
  R : Outport
  wires:
  IC/1 -> "[1.5 10]"/1
  "[1.5 10]"/1 -> Product2/1
  Product3/1 -> R/1
  Scale Factor/1 -> IC/1
  Product1/1 -> Product2/2
  Constant1/1 -> Product3/2
  Product2/1 -> Product3/1
  U_c/1 -> Product1/1, Product1/2

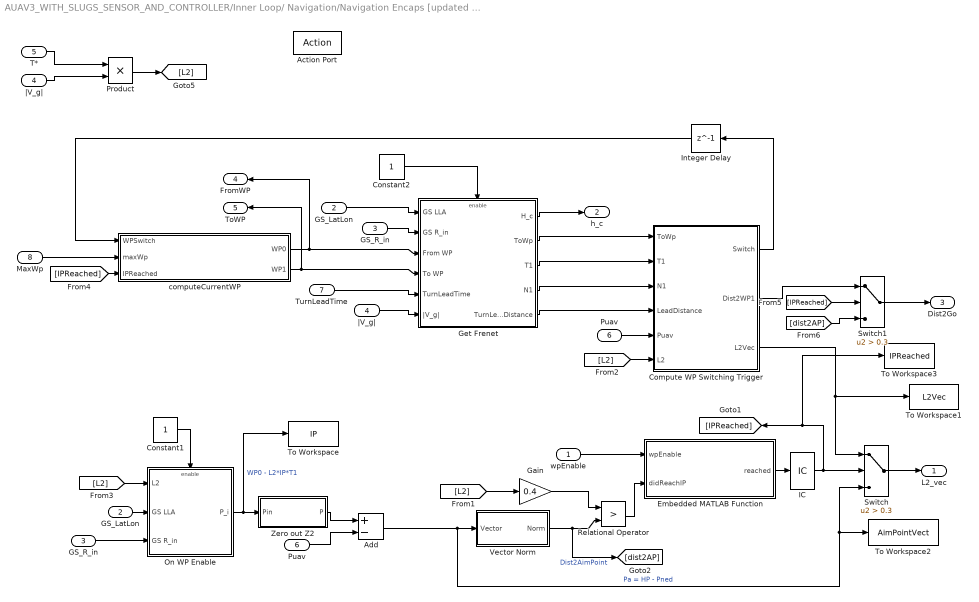
== system AUAV3_WITH_SLUGS_SENSOR_AND_CONTROLLER/Inner Loop/ Navigation/Navigation Encaps [updated 4.28.16]/Navigation/Normal WP  Navigation ==
  wpEnable : Inport
  GS_LatLon : Inport  Port=2
  GS_R_in : Inport  Port=3
  |V_g| : Inport  Port=4
  T* : Inport  Port=5
  Puav : Inport  Port=6
  TurnLeadTime : Inport  Port=7
  MaxWp : Inport  Port=8
  Action Port : ActionPort  ActionType=elseif
  Add : Sum  Inputs=+-
  Compute WP Switching Trigger : Subsystem
  Constant1 : Constant  OutDataTypeStr=boolean  SampleTime=0.01
  Constant2 : Constant  OutDataTypeStr=boolean  SampleTime=0.01
  Embedded MATLAB Function : MATLAB Function  TreatAsAtomicUnit=on
  "GS_LatLon " : InportShadow  Port=2
  "GS_R_in " : InportShadow  Port=3
  Gain : Gain  Gain=0.4
  Get Frenet : Subsystem
  IC : InitialCondition  Value=0
  Integer Delay : Delay  DelayLength=1  InitialCondition=1  InputProcessing=Inherited
  On WP Enable : Subsystem  TreatAsAtomicUnit=on
  Product : Product  OutDataTypeStr=single  RndMeth=Zero
  "Puav " : InportShadow  Port=6
  Relational Operator : RelationalOperator  Operator=>  OutDataTypeStr=boolean
  Switch : Switch  Criteria=u2 > Threshold  Threshold=0.3  ZeroCross=off
  Switch1 : Switch  Criteria=u2 > Threshold  Threshold=0.3  ZeroCross=off
  To Workspace : ToWorkspace  VariableName=IP  SampleTime=-1
  To Workspace1 : ToWorkspace  VariableName=L2Vec  SampleTime=-1
  To Workspace2 : ToWorkspace  VariableName=AimPointVect  SampleTime=-1
  To Workspace3 : ToWorkspace  VariableName=IPReached  SampleTime=-1
  Vector Norm : Subsystem  AncestorBlock=SLUGS_Library/Vector Norm
  Zero out Z2 : MATLAB Function  TreatAsAtomicUnit=on
  computeCurrentWP : MATLAB Function  TreatAsAtomicUnit=on
  "|V_g| " : InportShadow  Port=4
  L2_vec : Outport
  h_c : Outport  Port=2
  Dist2Go : Outport  Port=3
  FromWP : Outport  Port=4  InitialOutput=[1]
  ToWP : Outport  Port=5  InitialOutput=[2]
  wires:
  Get Frenet/1(H_c) -> h_c/1
  Constant2/1 -> Get Frenet/Enable
  Constant1/1 -> On WP Enable/Enable
  Integer Delay/1 -> computeCurrentWP/1(WPSwitch)
  [dist2AP] -> Switch1/3
  Switch1/1 -> Dist2Go/1
  Compute WP Switching Trigger/2(Dist2WP1) -> Switch1/1
  [IPReached] -> Switch1/2
  [IPReached] -> computeCurrentWP/3(IPReached)
  wpEnable/1 -> Embedded MATLAB Function/1(wpEnable)
  T*/1 -> Product/1
  |V_g|/1 -> Product/2
  Product/1 -> [L2]
  [L2] -> On WP Enable/1(L2)
  GS_LatLon/1 -> On WP Enable/2(GS LLA)
  GS_R_in/1 -> On WP Enable/3(GS R_in)
  On WP Enable/1(P_i) -> Zero out Z2/1(Pin), To Workspace/1  "WP0 - L2*IP*T1"
  Zero out Z2/1(P) -> Add/1
  Add/1 -> Vector Norm/1(Vector), Switch/3, To Workspace2/1  "Pa = HP - Pned"
  [L2] -> Gain/1
  Gain/1 -> Relational Operator/1
  Vector Norm/1(Norm) -> [dist2AP], Relational Operator/2  "Dist2AimPoint"
  Relational Operator/1 -> Embedded MATLAB Function/2(didReachIP)
  Switch/1 -> L2_vec/1
  Embedded MATLAB Function/1(reached) -> IC/1
  "GS_LatLon "/1 -> Get Frenet/1(GS LLA)
  "GS_R_in "/1 -> Get Frenet/2(GS R_in)
  Get Frenet/2(ToWp) -> Compute WP Switching Trigger/1(ToWp)
  Get Frenet/3(T1) -> Compute WP Switching Trigger/2(T1)
  Puav/1 -> Compute WP Switching Trigger/5(Puav)
  "Puav "/1 -> Add/2
  "|V_g| "/1 -> Get Frenet/6(|V_g|)
  TurnLeadTime/1 -> Get Frenet/5(TurnLeadTime)
  Get Frenet/5(TurnLeadDistance) -> Compute WP Switching Trigger/4(LeadDistance)
  Get Frenet/4(N1) -> Compute WP Switching Trigger/3(N1)
  Compute WP Switching Trigger/3(L2Vec) -> Switch/1, To Workspace1/1
  Compute WP Switching Trigger/1(Switch) -> Integer Delay/1
  computeCurrentWP/1(WP0) -> FromWP/1, Get Frenet/3(From WP)
  computeCurrentWP/2(WP1) -> ToWP/1, Get Frenet/4(To WP)
  MaxWp/1 -> computeCurrentWP/2(maxWp)
  [L2] -> Compute WP Switching Trigger/6(L2)
  IC/1 -> [IPReached], To Workspace3/1, Switch/2

== system AUAV3_WITH_SLUGS_SENSOR_AND_CONTROLLER/Inner Loop/ Navigation/Navigation Encaps [updated 4.28.16]/Navigation/RTB/Follow Mobile Navigation ==
  Mobile Location : Inport
  Follow Mobile? : Inport  Port=2
  MidLvl h_c : Inport  Port=3
  GS LatLon : Inport  Port=4
  GS R : Inport  Port=5
  Puav : Inport  Port=6
  Action Port : ActionPort  ActionType=then
  Compute Mobile Location : Subsystem  TreatAsAtomicUnit=on
  Constant : Constant  Value=[0 0 0]  OutDataTypeStr=single
  RTB : Constant  Value=0  OutDataTypeStr=uint8
  RTB1 : Constant  Value=0  OutDataTypeStr=uint8
  Simple Predictor : Subsystem
  Subtract : Sum  Inputs=+-
  Switch : Switch  Threshold=0.3
  To Workspace : ToWorkspace  VariableName=BP  SampleTime=-1
  Vector Norm : Subsystem  AncestorBlock=SLUGS_Library/Vector Norm
  Zero out Z1 : MATLAB Function  TreatAsAtomicUnit=on
  L2_vec : Outport
  h_c : Outport  Port=2
  Dist2Go : Outport  Port=3
  FromWP : Outport  Port=4  InitialOutput=[0]
  ToWP : Outport  Port=5  InitialOutput=[0]
  wires:
  RTB1/1 -> ToWP/1
  RTB/1 -> FromWP/1
  Vector Norm/1(Norm) -> Dist2Go/1
  Constant/1 -> Switch/3
  Compute Mobile Location/1(XYZ) -> Switch/1
  Follow Mobile?/1 -> Compute Mobile Location/Enable, Switch/2
  GS LatLon/1 -> Compute Mobile Location/2(GS LLA)
  GS R/1 -> Compute Mobile Location/3(GS R)
  Mobile Location/1 -> Compute Mobile Location/1("Lat, Lon")
  Simple Predictor/1(Predicted Bp) -> L2_vec/1
  Switch/1 -> Zero out Z1/1(Pin)
  Subtract/1 -> Vector Norm/1(Vector), Simple Predictor/1(Base Point), To Workspace/1
  Puav/1 -> Subtract/2
  Zero out Z1/1(P) -> Subtract/1
  MidLvl h_c/1 -> h_c/1

== system AUAV3_WITH_SLUGS_SENSOR_AND_CONTROLLER/Inner Loop/ Navigation/Navigation Encaps [updated 4.28.16]/Navigation/Recent Enable ==
  WP Fly : Inport
  Grab Upon Enable : Subsystem  TreatAsAtomicUnit=on
  IC1 : InitialCondition  Value=0
  IC2 : InitialCondition  Value=0
  IC3 : InitialCondition  Value=0
  IC4 : InitialCondition  Value=[36.988506 -122.055308]
  Subsystem : Subsystem
  WPEnable : Outport
  "GS, Lat Lon" : Outport  Port=2
  GS R_in : Outport  Port=3
  GS Alt (m) : Outport  Port=4
  wires:
  Grab Upon Enable/3(GS Altitude (m)) -> IC3/1
  IC2/1 -> Grab Upon Enable/Enable
  IC1/1 -> Subsystem/1(WP Fly)
  Subsystem/1(Just Enab) -> WPEnable/1, IC2/1
  WP Fly/1 -> IC1/1
  Grab Upon Enable/1("GS, Lon, Lat") -> IC4/1
  Grab Upon Enable/2(GS R_in) -> GS R_in/1
  IC4/1 -> "GS, Lat Lon"/1
  IC3/1 -> GS Alt (m)/1

== system AUAV3_WITH_SLUGS_SENSOR_AND_CONTROLLER/Position and Attitude Filter [updated 5.13.16]/Attitude Complimentary Filter COG/3D Filter/Filter1 ==
  In1 : Inport
  Discrete Zero-Pole : DiscreteZeroPole  Zeros=zerosd  Poles=polesd  Gain=gaind  SampleTime=SampleTime
  Out1 : Outport
  wires:
  Discrete Zero-Pole/1 -> Out1/1
  In1/1 -> Discrete Zero-Pole/1

== system AUAV3_WITH_SLUGS_SENSOR_AND_CONTROLLER/Position and Attitude Filter [updated 5.13.16]/Attitude Complimentary Filter COG/3D Filter/Filter2 ==
  In1 : Inport
  Discrete Zero-Pole : DiscreteZeroPole  Zeros=zerosd  Poles=polesd  Gain=gaind  SampleTime=SampleTime
  Out1 : Outport
  wires:
  In1/1 -> Discrete Zero-Pole/1
  Discrete Zero-Pole/1 -> Out1/1

== system AUAV3_WITH_SLUGS_SENSOR_AND_CONTROLLER/Position and Attitude Filter [updated 5.13.16]/Attitude Complimentary Filter COG/3D Filter/Filter3 ==
  In1 : Inport
  Discrete Zero-Pole : DiscreteZeroPole  Zeros=zerosd  Poles=polesd  Gain=gaind  SampleTime=SampleTime
  Out1 : Outport
  wires:
  Discrete Zero-Pole/1 -> Out1/1
  In1/1 -> Discrete Zero-Pole/1

== system AUAV3_WITH_SLUGS_SENSOR_AND_CONTROLLER/Position and Attitude Filter [updated 5.13.16]/Attitude Complimentary Filter COG/Normalize Vector1/Norm ==
  Vector : Inport
  Subsystem2 : Subsystem  AncestorBlock=SLUGS_Library/Subsystem1
  Subsystem3 : Subsystem  AncestorBlock=SLUGS_Library/Subsystem3
  Norm : Outport
  wires:
  Subsystem3/1(x dot y) -> Subsystem2/1(x)
  Vector/1 -> Subsystem3/2(y), Subsystem3/1(x)
  Subsystem2/1(sqrt(x)) -> Norm/1

== system AUAV3_WITH_SLUGS_SENSOR_AND_CONTROLLER/Position and Attitude Filter [updated 5.13.16]/Attitude Complimentary Filter COG/Normalize Vector2/Norm ==
  Vector : Inport
  Subsystem2 : Subsystem  AncestorBlock=SLUGS_Library/Subsystem1
  Subsystem3 : Subsystem  AncestorBlock=SLUGS_Library/Subsystem3
  Norm : Outport
  wires:
  Subsystem2/1(sqrt(x)) -> Norm/1
  Vector/1 -> Subsystem3/1(x), Subsystem3/2(y)
  Subsystem3/1(x dot y) -> Subsystem2/1(x)

== system AUAV3_WITH_SLUGS_SENSOR_AND_CONTROLLER/Position and Attitude Filter [updated 5.13.16]/Compute GS Location/Geod2ECEF1/eccentricity^2 ==
  " " : Product  OutDataTypeStr=single  SaturateOnIntegerOverflow=on  InputSameDT=on
  Re=equatorial radius1 : Constant  Value=Re  OutDataTypeStr=single
  Rp=polar radius : Constant  Value=Rp  OutDataTypeStr=single
  Sum5 : Sum  Inputs=|+-  SaturateOnIntegerOverflow=on  InputSameDT=on  OutDataTypeStr=Inherit: Same as first input
  const2 : Constant  OutDataTypeStr=single
  e^1 : Product  Inputs=*/  OutDataTypeStr=single  SaturateOnIntegerOverflow=on  InputSameDT=on
  e^2 : Outport
  wires:
  Sum5/1 -> e^2/1
  " "/1 -> Sum5/2
  e^1/1 -> " "/1, " "/2
  const2/1 -> Sum5/1
  Rp=polar radius/1 -> e^1/1
  Re=equatorial radius1/1 -> e^1/2

== system AUAV3_WITH_SLUGS_SENSOR_AND_CONTROLLER/Position and Attitude Filter [updated 5.13.16]/Geod2LTP1/ECEF2LTP (UEN)/From Body to Universal1 ==
  long : Inport
  lat : Inport  Port=2
  Mux : Mux  Inputs=2
  Reshape 9x1->3x1 : Reshape  OutputDimensionality=Customize  OutputDimensions=[3,3]
  Rotation Matrix from Long//Lat : Subsystem  mask(Vector Transformation){}
      mask help: Vector Transformation
      mask Display: disp('axis')
  DCM : Outport
  wires:
  Reshape 9x1->3x1/1 -> DCM/1
  Rotation Matrix from Long//Lat/1(DCM) -> Reshape 9x1->3x1/1
  Mux/1 -> Rotation Matrix from Long//Lat/1(long lat)
  long/1 -> Mux/1
  lat/1 -> Mux/2

== system AUAV3_WITH_SLUGS_SENSOR_AND_CONTROLLER/Position and Attitude Filter [updated 5.13.16]/Geod2LTP1/Geod2ECEF1/eccentricity^2 ==
  " " : Product  OutDataTypeStr=single  SaturateOnIntegerOverflow=on  InputSameDT=on
  Re=equatorial radius1 : Constant  Value=Re  OutDataTypeStr=single
  Rp=polar radius : Constant  Value=Rp  OutDataTypeStr=single
  Sum5 : Sum  Inputs=|+-  SaturateOnIntegerOverflow=on  InputSameDT=on  OutDataTypeStr=Inherit: Same as first input
  const2 : Constant  OutDataTypeStr=single
  e^1 : Product  Inputs=*/  OutDataTypeStr=single  SaturateOnIntegerOverflow=on  InputSameDT=on
  e^2 : Outport
  wires:
  Sum5/1 -> e^2/1
  " "/1 -> Sum5/2
  e^1/1 -> " "/1, " "/2
  const2/1 -> Sum5/1
  Rp=polar radius/1 -> e^1/1
  Re=equatorial radius1/1 -> e^1/2

== system AUAV3_WITH_SLUGS_SENSOR_AND_CONTROLLER/Position and Attitude Filter [updated 5.13.16]/Position Filter [updated 5.13.16]/BlendPosVel/2 FIlter Blend ==
  GPS_Z : Inport
  Baro_Alt : Inport  Port=2
  New GPS : Inport  Port=3
  baseHeight : Inport  Port=4
  Embedded MATLAB Function3 : MATLAB Function  TreatAsAtomicUnit=on
  Gain : Gain  Gain=1/(2*pi*baroCutoff)
  Sum : Sum  OutDataTypeStr=single
  "Tustin Lowpass,  Auto Initial Condition4" : Subsystem  mask(Tustin1stOrderLowpassAutoInitialCondition){f=baroCutoff, T=apSampleTime}
      mask prompts: f "Lowpass Frequency"; T "Sample Time"
      mask help: Takes a 3db rolloff frequency (in Hz, NOT radians/s) and a sample time. Performs a symbolic Tustin conversion and implements in a discrete filter. The initial output of the filter is set by the first sample.
      mask Help: Enter the desired 3db rolloff frequency in Hz and the sample time. Initial conditions are sampled automatically.
      mask Display: fprintf('%.2f Hz lowpass',f)
  Blend : Outport
  wires:
  Sum/1 -> "Tustin Lowpass,  Auto Initial Condition4"/1(In1)
  New GPS/1 -> Embedded MATLAB Function3/2(NewGPS)
  GPS_Z/1 -> Embedded MATLAB Function3/1(gps_h)
  baseHeight/1 -> Embedded MATLAB Function3/3(baseHeight)
  Embedded MATLAB Function3/1(h_rate) -> Gain/1
  "Tustin Lowpass,  Auto Initial Condition4"/1(Out1) -> Blend/1
  Gain/1 -> Sum/1
  Baro_Alt/1 -> Sum/2

== system AUAV3_WITH_SLUGS_SENSOR_AND_CONTROLLER/Position and Attitude Filter [updated 5.13.16]/Position Filter [updated 5.13.16]/BlendPosVel/3D Filter ==
  In1 : Inport
  Data Type Conversion1 : DataTypeConversion  OutDataTypeStr=single
  Data Type Conversion2 : DataTypeConversion  OutDataTypeStr=double
  Demux : Demux  Outputs=3
  Filter1 : Subsystem  mask(DiscretizedZeroPole){Zeros=zval, Poles=pval, Gain=kval, AbsTol=auto, SampleTime=TSample, method=tustin, Wc=1}
      mask prompts: Zeros "Zeros (enter in s-main:)"; Poles "Poles (enter in s-domain:)"; Gain "Gain (enter in s-domain:)"; AbsTol "Absolute tolerance:"; SampleTime "Sample time:"; Wc "Critical Frequency (Hz):"
      mask help: Continuous mask uses c2d to transform parameters onto the Discrete Zero-Pole block inside.
      mask init: same as AUAV3_WITH_SLUGS_SENSOR_AND_CONTROLLER/Position and Attitude Filter [updated 5.13.16]/Attitude Complimentary Filter COG/3D Filter/Filter1
      mask TypeOptions method: zoh | foh | tustin | prewarp | matched
      mask Callback method: hidecrit
      mask Display:
      | droots(zeross,poless,gainss)
      | text( 0.5, 1.0, method, 'verticalAlignment','top')
  Filter2 : Subsystem  mask(DiscretizedZeroPole){Zeros=zval, Poles=pval, Gain=kval, AbsTol=auto, SampleTime=TSample, method=tustin, Wc=1}
      mask prompts: Zeros "Zeros (enter in s-main:)"; Poles "Poles (enter in s-domain:)"; Gain "Gain (enter in s-domain:)"; AbsTol "Absolute tolerance:"; SampleTime "Sample time:"; Wc "Critical Frequency (Hz):"
      mask help: Continuous mask uses c2d to transform parameters onto the Discrete Zero-Pole block inside.
      mask init: same as AUAV3_WITH_SLUGS_SENSOR_AND_CONTROLLER/Position and Attitude Filter [updated 5.13.16]/Attitude Complimentary Filter COG/3D Filter/Filter1
      mask TypeOptions method: zoh | foh | tustin | prewarp | matched
      mask Callback method: hidecrit
      mask Display:
      | droots(zeross,poless,gainss)
      | text( 0.5, 1.0, method, 'verticalAlignment','top')
  Filter3 : Subsystem  mask(DiscretizedZeroPole){Zeros=zval, Poles=pval, Gain=kval, AbsTol=auto, SampleTime=TSample, method=tustin, Wc=1}
      mask prompts: Zeros "Zeros (enter in s-main:)"; Poles "Poles (enter in s-domain:)"; Gain "Gain (enter in s-domain:)"; AbsTol "Absolute tolerance:"; SampleTime "Sample time:"; Wc "Critical Frequency (Hz):"
      mask help: Continuous mask uses c2d to transform parameters onto the Discrete Zero-Pole block inside.
      mask init: same as AUAV3_WITH_SLUGS_SENSOR_AND_CONTROLLER/Position and Attitude Filter [updated 5.13.16]/Attitude Complimentary Filter COG/3D Filter/Filter1
      mask TypeOptions method: zoh | foh | tustin | prewarp | matched
      mask Callback method: hidecrit
      mask Display:
      | droots(zeross,poless,gainss)
      | text( 0.5, 1.0, method, 'verticalAlignment','top')
  myMux Fun1 : MATLAB Function  TreatAsAtomicUnit=on
  Out1 : Outport
  wires:
  Data Type Conversion1/1 -> Out1/1
  Data Type Conversion2/1 -> Demux/1
  Demux/1 -> Filter1/1(In1)
  Demux/2 -> Filter2/1(In1)
  Demux/3 -> Filter3/1(In1)
  Filter1/1(Out1) -> myMux Fun1/1(u1)
  Filter2/1(Out1) -> myMux Fun1/2(u2)
  Filter3/1(Out1) -> myMux Fun1/3(u3)
  In1/1 -> Data Type Conversion2/1
  myMux Fun1/1(y) -> Data Type Conversion1/1

== system AUAV3_WITH_SLUGS_SENSOR_AND_CONTROLLER/Position and Attitude Filter [updated 5.13.16]/Position Filter [updated 5.13.16]/BlendPosVel/CompFiltRate ==
  Rate : Inport
  LoPass : Inport  Port=2
  1D Filter1 : Subsystem  RTWFcnName=TustinFilter3D  mask{zval=[], pval=[0], kval=1, TSample=T}
      mask prompts: zval "Zeros"; pval "Poles"; kval "Gains"; TSample "Sample Time"
      settings: RTWFcnNameOpts=User specified  RTWFileNameOpts=Use function name
      mask Display:
      | droots(zval,pval,kval)
      | port_label('input',1,'1D')
  Gain : Gain  Gain=omega
  Sum : Sum  Inputs=++|
  Sum1 : Sum  Inputs=|+-
  Unit Delay : UnitDelay  SampleTime=T
  Blend : Outport
  wires:
  Unit Delay/1 -> Sum1/2
  LoPass/1 -> Sum1/1
  Sum1/1 -> Gain/1
  Gain/1 -> Sum/2
  Rate/1 -> Sum/1
  Sum/1 -> 1D Filter1/1(In1)
  1D Filter1/1(Out1) -> Unit Delay/1, Blend/1

== system AUAV3_WITH_SLUGS_SENSOR_AND_CONTROLLER/Position and Attitude Filter [updated 5.13.16]/Position Filter [updated 5.13.16]/BlendPosVel/CompFiltRate1 ==
  Rate : Inport
  LoPass : Inport  Port=2
  1D Filter1 : Subsystem  RTWFcnName=TustinFilter3D  mask{zval=[], pval=[0], kval=1, TSample=T}
      mask prompts: zval "Zeros"; pval "Poles"; kval "Gains"; TSample "Sample Time"
      settings: RTWFcnNameOpts=User specified  RTWFileNameOpts=Use function name
      mask Display:
      | droots(zval,pval,kval)
      | port_label('input',1,'1D')
  Gain : Gain  Gain=omega
  Sum : Sum  Inputs=++|
  Sum1 : Sum  Inputs=|+-
  Unit Delay : UnitDelay  SampleTime=T
  Blend : Outport
  wires:
  Unit Delay/1 -> Sum1/2
  LoPass/1 -> Sum1/1
  Sum1/1 -> Gain/1
  Gain/1 -> Sum/2
  Rate/1 -> Sum/1
  Sum/1 -> 1D Filter1/1(In1)
  1D Filter1/1(Out1) -> Unit Delay/1, Blend/1
